simulink model "pend_est_c"  (Simulink 5.0)
settings: Solver=ode45  StartTime=0.0  StopTime=10.0  RelTol=1e-3
values from neighbouring files (symbols this model uses):
  A = zeros(4); A(1,3) = 1; A(2,4) = 1    [pend_model.m]    (also in pr_400.m = [1 1; 1 1])
  B = zeros(4,1); B(3) = alpha1*delta; B(4) = -alpha1*beta    [pend_model.m]
  C = [1 0 0 0; 0 1 0 0]    [trash.m]
  D = [0;0]    [trash.m]
  Ts = 0.01    [trash.m]
undefined symbols (not defined in the file or in its folder): Ac, Bc, Cc, Dc
settings Model: Creator=kannan  LastModifiedBy=kannanm  ExtModeAutoUpdateStatusClock=off

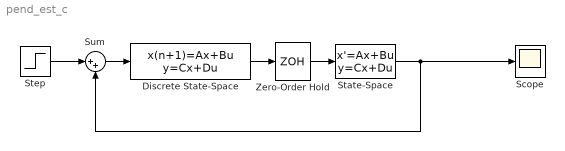
== system pend_est_c ==
  Discrete State-Space : DiscreteStateSpace  A=Ac  B=Bc  C=Cc  D=Dc  X0=[0 0 0 0]  SampleTime=Ts
  Scope : Scope
  State-Space : StateSpace  A=A  B=B  C=C  D=D  X0=[0 0.01 0 0]
  Step : Step  After=0  SampleTime=Ts
  Sum : Sum  Inputs=|++  SaturateOnIntegerOverflow=on
  Zero-Order Hold : ZeroOrderHold  SampleTime=Ts
  wires:
  Step/1 -> Sum/1
  State-Space/1 -> Scope/1, Sum/2
  Zero-Order Hold/1 -> State-Space/1
  Sum/1 -> Discrete State-Space/1
  Discrete State-Space/1 -> Zero-Order Hold/1
